simulink model "motor_fault_detection_main"  (R2018a)
settings: Solver=ode2  StartTime=0.0  StopTime=5.0  FixedStep=1e-5  RelTol=1e-3
libraries: powerlib x4
settings Model: Creator=FAVOUR PC  LastModifiedBy=FAVOUR PC
settings SolverCC: PositivePriorityOrder=on

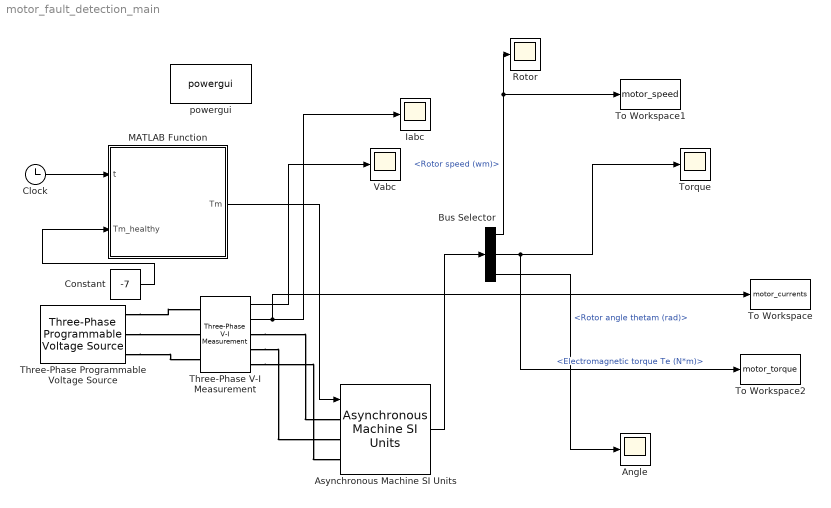
== system motor_fault_detection_main ==
  "Angle " : Scope
  Asynchronous Machine SI Units : powerlib/Machines/Asynchronous Machine SI Units  RotorType=Squirrel-cage  PresetModel=No  MechanicalLoad=Torque Tm  ShowDetailedParameters=on  ReferenceFrame=Stationary  Units=SI  MeasurementBus=off  NominalParameters=[5500 400 50]  Stator=[1.405 0.005839]  Rotor=[1.395 0.005839]  Cage1=[0.4155 0.002066]  Cage2=[0.4168 0.0003495]  Lm=0.1722  Mechanical=[0.0131 0.05 2]  PolePairs=2  InitialConditions=[0 0 0 0 0 0 0 0]  SimulateSaturation=off  Saturation=[14.03593122, 27.81365428, 53.79336849, 72.68890987, 97.98006896, 148.6815601, 215.7428561, 302.9841135, 428.7778367 ; 230, 322, 414, 460, 506, 552, 598, 644, 690]  LoadFlowParameters=1492000  TsPowergui=0  TsBlock=-1  IterativeModel=Trapezoidal non iterative  IterativeDiscreteModel=Trapezoidal non iterative  Pmec=1.492e+006
  Bus Selector : BusSelector  OutputSignals=Mechanical.Rotor speed (wm),Mechanical.Electromagnetic torque Te (N*m),Mechanical.Rotor angle thetam (rad)
  Clock : Clock
  Constant : Constant  Value=-7
  "Iabc " : Scope
  MATLAB Function : MATLAB Function  TreatAsAtomicUnit=on
  "Rotor " : Scope
  Three-Phase Programmable Voltage Source : powerlib/Electrical Sources/Three-Phase Programmable Voltage Source  PositiveSequence="[100  0 60]"  VariationEntity=None  VariationType=Table of time-amplitude pairs  VariationTypeAlt=Step  VariationStep=0.5  VariationRate=10  VariationMagnitude=0.3  VariationFrequency=2  VariationTiming=[1 2]  VariationPhaseA=off  Amplitudes=[1 0.8 1.2 1.0]  TimeValues=[0 0.1 0.15 0.2]  HarmonicGeneration=off  HarmonicA=[3 0.2 -25 0]  HarmonicB=[2 0.15 35 2]  Timing="[0.05  3]"  BusType=swing  Pref=0  Qref=0  Qmin=-inf  Qmax=inf
  Three-Phase V-I Measurement : powerlib/Measurements/Three-Phase V-I Measurement  VoltageMeasurement=phase-to-phase  SetLabelV=off  LabelV=Vabc  Vpu=off  VpuLL=off  CurrentMeasurement=yes  SetLabelI=off  LabelI=Iabc  Ipu=off  Pbase=100e6  Vbase=500e3  OutputType=Complex  PhasorSimulation=off  PSBequivalent=0
  To Workspace : ToWorkspace  VariableName=motor_currents  SaveFormat=Structure With Time  SampleTime=-1
  To Workspace1 : ToWorkspace  VariableName=motor_speed  SaveFormat=Structure With Time  SampleTime=-1
  To Workspace2 : ToWorkspace  VariableName=motor_torque  SaveFormat=Structure With Time  SampleTime=-1
  "Torque " : Scope
  "Vabc " : Scope
  powergui : powerlib/powergui  Priority=1  SimulationMode=Discrete  SampleTime=1e-5  frequency=60  Iterations=50  frequencyindice=50  Pbase=100e6  ErrMax=1e-4  UnitsV=kV  UnitsW=MW  buscounter=0  FunctionMessages=off  echomessages=off  EnableUseOfTLC=off  CurrentSourceSwitches=off  DisableSnubberDevices=off  DisableRonSwitches=off  DisableVfSwitches=off  DisplayEquations=off  SolverType=Tustin/Backward Euler (TBE)  Interpol=off  ExternalGateDelay=off  methode=off  Ts=100  x0status=blocks  SPID=on  SwTol=0  HookPort=off  RestoreLinks=warning  ResistiveCurrentMeasurement=off  Frange=[0:2:500]  Ylog=off  Xlog=on  ShowGrid=off  save=off  variable=ZData  structure=0  ZoomFFT=off  StartTime=0.0  cycles=1  DisplayStyle=1  fundamental=60  FreqAxis=off  MaxFrequency=1000  frequencyindicesteady=1  RmsSteady=1  display=off
  wires:
  Asynchronous Machine SI Units/1 -> Bus Selector/1
  Three-Phase V-I Measurement/2 -> To Workspace/1, "Iabc "/1
  Bus Selector/1 -> To Workspace1/1, "Rotor "/1  "<Rotor speed (wm)>"
  Bus Selector/2 -> "Torque "/1, To Workspace2/1  "<Electromagnetic torque Te (N*m)>"
  Three-Phase V-I Measurement/1 -> "Vabc "/1
  Bus Selector/3 -> "Angle "/1  "<Rotor angle thetam (rad)>"
  MATLAB Function/1(Tm) -> Asynchronous Machine SI Units/1
  Constant/1 -> MATLAB Function/2(Tm_healthy)
  Clock/1 -> MATLAB Function/1(t)
  connections:
  Three-Phase Programmable Voltage Source/RConn1 -- Three-Phase V-I Measurement/LConn1
  Three-Phase Programmable Voltage Source/RConn2 -- Three-Phase V-I Measurement/LConn2
  Three-Phase Programmable Voltage Source/RConn3 -- Three-Phase V-I Measurement/LConn3
  Three-Phase V-I Measurement/RConn1 -- Asynchronous Machine SI Units/LConn1
  Three-Phase V-I Measurement/RConn2 -- Asynchronous Machine SI Units/LConn2
  Three-Phase V-I Measurement/RConn3 -- Asynchronous Machine SI Units/LConn3

== matlab function motor_fault_detection_main/MATLAB Function ==
  data: t input; Tm output; Tm_healthy input
function Tm = bearingFault(t, Tm_healthy)
    % Bearing fault parameters - REDUCED FREQUENCY
    fault_start = 2;        
    bearing_freq = 10;      % Reduced to 10 Hz for visibility
    severity = 0.3;         % 30% severity
    
    % Normal operation before fault
    if t < fault_start
        Tm = Tm_healthy;
        return;
    end
    
    % Time since fault started
    t_fault = t - fault_start;
    
    % Create periodic impulses - more pronounced
    fault_period = 1/bearing_freq;
    phase = mod(t_fault, fault_period);
    
    % Create impulse train (20% duty cycle)
    if phase < 0.2 * fault_period
        % During impulse
        impulse_amplitude = severity * abs(Tm_healthy);
        Tm = Tm_healthy - impulse_amplitude;
    else
        % Normal torque
        Tm = Tm_healthy;
    end
end
